simulink model "test_mdl1"  (R2023a)
settings: Solver=VariableStepAuto  StartTime=0.0  StopTime=10.0  RelTol=1e-3
(part 7 of 8)

== system test_mdl1/VehicleCAN/PCM/PowertrainData_6 ==
  BrkTot_Tq_RqFapLc : Constant  Value=0
  FapLc_B_Err : Constant  Value=0
  TrnAin_Pc_RqDrv : Constant  Value=0
  bus_creator : BusCreator  Inputs=3
  out_port : Outport
  wires:
  bus_creator/1 -> out_port/1  "test_mdl1"
  BrkTot_Tq_RqFapLc/1 -> bus_creator/1  "BrkTot_Tq_RqFapLc"
  FapLc_B_Err/1 -> bus_creator/2  "FapLc_B_Err"
  TrnAin_Pc_RqDrv/1 -> bus_creator/3  "TrnAin_Pc_RqDrv"

== system test_mdl1/VehicleCAN/PCM/PowertrainData_7 ==
  EcoCochA_Pc_Dsply : Constant  Value=0
  EcoCochCrus_Pc_Dsply : Constant  Value=0
  EcoCochDecel_Pc_Dsply : Constant  Value=0
  EcoCochIdlFuel_Pc_Dsply : Constant  Value=0
  EcoCochInstNeg_B_Dsply : Constant  Value=0
  EcoCochInst_Pc_Dsply : Constant  Value=0
  EcoCochShif_Pc_Dsply : Constant  Value=0
  bus_creator : BusCreator  Inputs=7
  out_port : Outport
  wires:
  bus_creator/1 -> out_port/1  "test_mdl1"
  EcoCochA_Pc_Dsply/1 -> bus_creator/1  "EcoCochA_Pc_Dsply"
  EcoCochCrus_Pc_Dsply/1 -> bus_creator/2  "EcoCochCrus_Pc_Dsply"
  EcoCochDecel_Pc_Dsply/1 -> bus_creator/3  "EcoCochDecel_Pc_Dsply"
  EcoCochIdlFuel_Pc_Dsply/1 -> bus_creator/4  "EcoCochIdlFuel_Pc_Dsply"
  EcoCochInstNeg_B_Dsply/1 -> bus_creator/5  "EcoCochInstNeg_B_Dsply"
  EcoCochInst_Pc_Dsply/1 -> bus_creator/6  "EcoCochInst_Pc_Dsply"
  EcoCochShif_Pc_Dsply/1 -> bus_creator/7  "EcoCochShif_Pc_Dsply"

== system test_mdl1/VehicleCAN/PCM/PowertrainData_9 ==
  AutoTowActv_B_Stat : Constant  Value=0
  AutoTowAllw_D_StatMnu : Constant  Value=0
  EngExhMdeQuiet_D2_Stat : Constant  Value=0
  GrossTrainWeight_M_Est : Constant  Value=0
  HvacCmprLim_D_Stat : Constant  Value=0
  TrailCtlPt_B_Falt : Constant  Value=0
  Veh_V_DsplyTrailCtlSet : Constant  Value=0
  WakeAlarm1_B_Typ : Constant  Value=0
  WakeAlarm1_T_Rq : Constant  Value=0
  bus_creator : BusCreator  Inputs=9
  out_port : Outport
  wires:
  bus_creator/1 -> out_port/1  "test_mdl1"
  AutoTowActv_B_Stat/1 -> bus_creator/1  "AutoTowActv_B_Stat"
  AutoTowAllw_D_StatMnu/1 -> bus_creator/2  "AutoTowAllw_D_StatMnu"
  EngExhMdeQuiet_D2_Stat/1 -> bus_creator/3  "EngExhMdeQuiet_D2_Stat"
  GrossTrainWeight_M_Est/1 -> bus_creator/4  "GrossTrainWeight_M_Est"
  HvacCmprLim_D_Stat/1 -> bus_creator/5  "HvacCmprLim_D_Stat"
  TrailCtlPt_B_Falt/1 -> bus_creator/6  "TrailCtlPt_B_Falt"
  Veh_V_DsplyTrailCtlSet/1 -> bus_creator/7  "Veh_V_DsplyTrailCtlSet"
  WakeAlarm1_B_Typ/1 -> bus_creator/8  "WakeAlarm1_B_Typ"
  WakeAlarm1_T_Rq/1 -> bus_creator/9  "WakeAlarm1_T_Rq"

== system test_mdl1/VehicleCAN/PCM/Powertrain_Data_4 ==
  BpedDrvMsgTxt_B_Dsply : Constant  Value=0
  FuelLvlWarn_D_ActlEng : Constant  Value=0
  FuelLvl_Pc_DsplyEng : Constant  Value=0
  FuelRange_L_DsplyEng : Constant  Value=0
  RearDiffOilTeWarn_B_Rq : Constant  Value=0
  RearDiffOil_Te_Actl : Constant  Value=0
  SelDrvMdePt_D_Stat : Constant  Value=0
  bus_creator : BusCreator  Inputs=7
  out_port : Outport
  wires:
  bus_creator/1 -> out_port/1  "test_mdl1"
  BpedDrvMsgTxt_B_Dsply/1 -> bus_creator/1  "BpedDrvMsgTxt_B_Dsply"
  FuelLvlWarn_D_ActlEng/1 -> bus_creator/2  "FuelLvlWarn_D_ActlEng"
  FuelLvl_Pc_DsplyEng/1 -> bus_creator/3  "FuelLvl_Pc_DsplyEng"
  FuelRange_L_DsplyEng/1 -> bus_creator/4  "FuelRange_L_DsplyEng"
  RearDiffOilTeWarn_B_Rq/1 -> bus_creator/5  "RearDiffOilTeWarn_B_Rq"
  RearDiffOil_Te_Actl/1 -> bus_creator/6  "RearDiffOil_Te_Actl"
  SelDrvMdePt_D_Stat/1 -> bus_creator/7  "SelDrvMdePt_D_Stat"

== system test_mdl1/VehicleCAN/PCM/Powertrain_Data_5 ==
  AdasLcObtclAbrt_B_Stat : Constant  Value=0
  AirDamPos_D_Stat : Constant  Value=0
  BattRgenLoChrg_D_RqEng : Constant  Value=0
  BattRgenLoDChrg_D_RqEng : Constant  Value=0
  FapLcActv_B_Stat : Constant  Value=0
  FapLcInhbt_B_Rq : Constant  Value=0
  FapLcMaxGrdAbrt_B_Stat : Constant  Value=0
  FapLcMaxGrdInhbt_B_Stat : Constant  Value=0
  FapLcObstcl_B_Stat : Constant  Value=0
  FapLcPrchgBrk_B_Rq : Constant  Value=0
  FapLcStopHold_B_Rq : Constant  Value=0
  bus_creator : BusCreator  Inputs=11
  out_port : Outport
  wires:
  bus_creator/1 -> out_port/1  "test_mdl1"
  AdasLcObtclAbrt_B_Stat/1 -> bus_creator/1  "AdasLcObtclAbrt_B_Stat"
  AirDamPos_D_Stat/1 -> bus_creator/2  "AirDamPos_D_Stat"
  BattRgenLoChrg_D_RqEng/1 -> bus_creator/3  "BattRgenLoChrg_D_RqEng"
  BattRgenLoDChrg_D_RqEng/1 -> bus_creator/4  "BattRgenLoDChrg_D_RqEng"
  FapLcActv_B_Stat/1 -> bus_creator/5  "FapLcActv_B_Stat"
  FapLcInhbt_B_Rq/1 -> bus_creator/6  "FapLcInhbt_B_Rq"
  FapLcMaxGrdAbrt_B_Stat/1 -> bus_creator/7  "FapLcMaxGrdAbrt_B_Stat"
  FapLcMaxGrdInhbt_B_Stat/1 -> bus_creator/8  "FapLcMaxGrdInhbt_B_Stat"
  FapLcObstcl_B_Stat/1 -> bus_creator/9  "FapLcObstcl_B_Stat"
  FapLcPrchgBrk_B_Rq/1 -> bus_creator/10  "FapLcPrchgBrk_B_Rq"
  FapLcStopHold_B_Rq/1 -> bus_creator/11  "FapLcStopHold_B_Rq"

== system test_mdl1/VehicleCAN/PCM/Stop_Start ==
  AutoStopPtDelta_I_Est : Constant  Value=0
  HiElPwInhbt_B_Stat : Constant  Value=0
  OdoTripVerify_L_Actl : Constant  Value=0
  StopStrtDrvMde_D_Indic : Constant  Value=0
  StopStrtIODTxt_D_Rq : Constant  Value=0
  StopStrtMsgTxt_D_Rq : Constant  Value=0
  StopStrtStdby_D_Indic : Constant  Value=0
  bus_creator : BusCreator  Inputs=7
  out_port : Outport
  wires:
  bus_creator/1 -> out_port/1  "test_mdl1"
  AutoStopPtDelta_I_Est/1 -> bus_creator/1  "AutoStopPtDelta_I_Est"
  HiElPwInhbt_B_Stat/1 -> bus_creator/2  "HiElPwInhbt_B_Stat"
  OdoTripVerify_L_Actl/1 -> bus_creator/3  "OdoTripVerify_L_Actl"
  StopStrtDrvMde_D_Indic/1 -> bus_creator/4  "StopStrtDrvMde_D_Indic"
  StopStrtIODTxt_D_Rq/1 -> bus_creator/5  "StopStrtIODTxt_D_Rq"
  StopStrtMsgTxt_D_Rq/1 -> bus_creator/6  "StopStrtMsgTxt_D_Rq"
  StopStrtStdby_D_Indic/1 -> bus_creator/7  "StopStrtStdby_D_Indic"

== system test_mdl1/VehicleCAN/PCM/TesterPhysicalResPCM ==
  TesterPhysicalResPCM : Constant  Value=0
  bus_creator : BusCreator  Inputs=1
  out_port : Outport
  wires:
  bus_creator/1 -> out_port/1  "test_mdl1"
  TesterPhysicalResPCM/1 -> bus_creator/1  "TesterPhysicalResPCM"

== system test_mdl1/VehicleCAN/PCM/TorqueDataEngFlags ==
  PrplWhlTotTqRq_No_Cnt : Constant  Value=0
  PrplWhlTotTqRq_No_Cs : Constant  Value=0
  PrplWhlTot_Tq_LimMn : Constant  Value=0
  PrplWhlTot_Tq_Rq : Constant  Value=0
  PtDrvMde_D_Stat : Constant  Value=0
  bus_creator : BusCreator  Inputs=5
  out_port : Outport
  wires:
  bus_creator/1 -> out_port/1  "test_mdl1"
  PrplWhlTotTqRq_No_Cnt/1 -> bus_creator/1  "PrplWhlTotTqRq_No_Cnt"
  PrplWhlTotTqRq_No_Cs/1 -> bus_creator/2  "PrplWhlTotTqRq_No_Cs"
  PrplWhlTot_Tq_LimMn/1 -> bus_creator/3  "PrplWhlTot_Tq_LimMn"
  PrplWhlTot_Tq_Rq/1 -> bus_creator/4  "PrplWhlTot_Tq_Rq"
  PtDrvMde_D_Stat/1 -> bus_creator/5  "PtDrvMde_D_Stat"

== system test_mdl1/VehicleCAN/PCM/TransGearData ==
  GboxOil_Te_Actl : Constant  Value=0
  GearLvrPos_D_Actl : Constant  Value=0
  SelDrvMdeSwtch_D_Stat3 : Constant  Value=0
  TrnShifActv_B_Actl : Constant  Value=0
  TrnSrvcRqd_B_Rq : Constant  Value=0
  bus_creator : BusCreator  Inputs=5
  out_port : Outport
  wires:
  bus_creator/1 -> out_port/1  "test_mdl1"
  GboxOil_Te_Actl/1 -> bus_creator/1  "GboxOil_Te_Actl"
  GearLvrPos_D_Actl/1 -> bus_creator/2  "GearLvrPos_D_Actl"
  SelDrvMdeSwtch_D_Stat3/1 -> bus_creator/3  "SelDrvMdeSwtch_D_Stat3"
  TrnShifActv_B_Actl/1 -> bus_creator/4  "TrnShifActv_B_Actl"
  TrnSrvcRqd_B_Rq/1 -> bus_creator/5  "TrnSrvcRqd_B_Rq"

== system test_mdl1/VehicleCAN/PCM/VehicleOperatingModes ==
  ElPw_D_Stat : Constant  Value=0
  ElPw_D_StatStrtStop : Constant  Value=0
  Eng_D_Stat : Constant  Value=0
  PlgActvArb_B_Actl : Constant  Value=0
  PrplWhlRgenMn_Tq_Actl : Constant  Value=0
  PrplWhlTot2_Tq_Actl : Constant  Value=0
  PwPckTq_D_Stat : Constant  Value=0
  TrnAinTq_D_Qf : Constant  Value=0
  TrnAin_Tq_Actl : Constant  Value=0
  bus_creator : BusCreator  Inputs=9
  out_port : Outport
  wires:
  bus_creator/1 -> out_port/1  "test_mdl1"
  ElPw_D_Stat/1 -> bus_creator/1  "ElPw_D_Stat"
  ElPw_D_StatStrtStop/1 -> bus_creator/2  "ElPw_D_StatStrtStop"
  Eng_D_Stat/1 -> bus_creator/3  "Eng_D_Stat"
  PlgActvArb_B_Actl/1 -> bus_creator/4  "PlgActvArb_B_Actl"
  PrplWhlRgenMn_Tq_Actl/1 -> bus_creator/5  "PrplWhlRgenMn_Tq_Actl"
  PrplWhlTot2_Tq_Actl/1 -> bus_creator/6  "PrplWhlTot2_Tq_Actl"
  PwPckTq_D_Stat/1 -> bus_creator/7  "PwPckTq_D_Stat"
  TrnAinTq_D_Qf/1 -> bus_creator/8  "TrnAinTq_D_Qf"
  TrnAin_Tq_Actl/1 -> bus_creator/9  "TrnAin_Tq_Actl"

== system test_mdl1/VehicleCAN/PCM_HEV/Cluster_HEV_Data10_FD1 ==
  Rng%ChrgAvg_L_Dsply : Constant  Value=0
  bus_creator : BusCreator  Inputs=1
  out_port : Outport
  wires:
  bus_creator/1 -> out_port/1  "test_mdl1"
  Rng%ChrgAvg_L_Dsply/1 -> bus_creator/1  "Rng%ChrgAvg_L_Dsply"

== system test_mdl1/VehicleCAN/PCM_HEV/Cluster_HEV_Data1_FD1 ==
  ChrgStat_D_Dsply : Constant  Value=0
  RgenTrip_L_Dsply : Constant  Value=0
  RgenTrip_Pc_Dsply : Constant  Value=0
  bus_creator : BusCreator  Inputs=3
  out_port : Outport
  wires:
  bus_creator/1 -> out_port/1  "test_mdl1"
  ChrgStat_D_Dsply/1 -> bus_creator/1  "ChrgStat_D_Dsply"
  RgenTrip_L_Dsply/1 -> bus_creator/2  "RgenTrip_L_Dsply"
  RgenTrip_Pc_Dsply/1 -> bus_creator/3  "RgenTrip_Pc_Dsply"

== system test_mdl1/VehicleCAN/PCM_HEV/Cluster_HEV_Data2 ==
  EffWhlLvl2_Pc_Dsply : Constant  Value=0
  EffWhlThresOn_B_Dsply : Constant  Value=0
  EffWhlThres_Pc_Dsply : Constant  Value=0
  EngActv_B_Dsply : Constant  Value=0
  EngOnMsg1_D_Dsply : Constant  Value=0
  EngOnMsg2_D_Dsply : Constant  Value=0
  EngPwLvl_Pc_Dsply : Constant  Value=0
  FuelMaintMde_D_Dsply : Constant  Value=0
  PwrFlowTxt_D_Dsply : Constant  Value=0
  bus_creator : BusCreator  Inputs=9
  out_port : Outport
  wires:
  bus_creator/1 -> out_port/1  "test_mdl1"
  EffWhlLvl2_Pc_Dsply/1 -> bus_creator/1  "EffWhlLvl2_Pc_Dsply"
  EffWhlThresOn_B_Dsply/1 -> bus_creator/2  "EffWhlThresOn_B_Dsply"
  EffWhlThres_Pc_Dsply/1 -> bus_creator/3  "EffWhlThres_Pc_Dsply"
  EngActv_B_Dsply/1 -> bus_creator/4  "EngActv_B_Dsply"
  EngOnMsg1_D_Dsply/1 -> bus_creator/5  "EngOnMsg1_D_Dsply"
  EngOnMsg2_D_Dsply/1 -> bus_creator/6  "EngOnMsg2_D_Dsply"
  EngPwLvl_Pc_Dsply/1 -> bus_creator/7  "EngPwLvl_Pc_Dsply"
  FuelMaintMde_D_Dsply/1 -> bus_creator/8  "FuelMaintMde_D_Dsply"
  PwrFlowTxt_D_Dsply/1 -> bus_creator/9  "PwrFlowTxt_D_Dsply"

== system test_mdl1/VehicleCAN/PCM_HEV/Cluster_HEV_Data3_FD1 ==
  EffRgenThres_Pc_Dsply : Constant  Value=0
  EngMdeMsgTxt_D_Rq : Constant  Value=0
  Rng%ChrgInst_L_Dsply : Constant  Value=0
  bus_creator : BusCreator  Inputs=3
  out_port : Outport
  wires:
  bus_creator/1 -> out_port/1  "test_mdl1"
  EffRgenThres_Pc_Dsply/1 -> bus_creator/1  "EffRgenThres_Pc_Dsply"
  EngMdeMsgTxt_D_Rq/1 -> bus_creator/2  "EngMdeMsgTxt_D_Rq"
  Rng%ChrgInst_L_Dsply/1 -> bus_creator/3  "Rng%ChrgInst_L_Dsply"

== system test_mdl1/VehicleCAN/PCM_HEV/Cluster_HEV_Data5 ==
  HybMdeStat_D_Dsply : Constant  Value=0
  PlgActvArb_B_Dsply : Constant  Value=0
  bus_creator : BusCreator  Inputs=2
  out_port : Outport
  wires:
  bus_creator/1 -> out_port/1  "test_mdl1"
  HybMdeStat_D_Dsply/1 -> bus_creator/1  "HybMdeStat_D_Dsply"
  PlgActvArb_B_Dsply/1 -> bus_creator/2  "PlgActvArb_B_Dsply"

== system test_mdl1/VehicleCAN/PCM_HEV/DCACA_Data4 ==
  DcacElPw_D_Stat : Constant  Value=0
  DcacEngOnMsgTxt_D_Rq : Constant  Value=0
  DcacFaltMsgTxt_D_Rq : Constant  Value=0
  DcacGfciTest_B_Rq : Constant  Value=0
  DcacHw_D_Confg : Constant  Value=0
  DcacLedCtl_D_Rq : Constant  Value=0
  DcacLoFuelMsgTxt_D_Rq : Constant  Value=0
  DcacOn_B_Rq : Constant  Value=0
  DcacOut1_Pw_Dsply : Constant  Value=0
  DcacOut2_Pw_Dsply : Constant  Value=0
  DcacOut_Pw_DsplyMx : Constant  Value=0
  DcacSys_B_Falt : Constant  Value=0
  PwBedPnlEnbl_B_Rq : Constant  Value=0
  bus_creator : BusCreator  Inputs=13
  out_port : Outport
  wires:
  bus_creator/1 -> out_port/1  "test_mdl1"
  DcacElPw_D_Stat/1 -> bus_creator/1  "DcacElPw_D_Stat"
  DcacEngOnMsgTxt_D_Rq/1 -> bus_creator/2  "DcacEngOnMsgTxt_D_Rq"
  DcacFaltMsgTxt_D_Rq/1 -> bus_creator/3  "DcacFaltMsgTxt_D_Rq"
  DcacGfciTest_B_Rq/1 -> bus_creator/4  "DcacGfciTest_B_Rq"
  DcacHw_D_Confg/1 -> bus_creator/5  "DcacHw_D_Confg"
  DcacLedCtl_D_Rq/1 -> bus_creator/6  "DcacLedCtl_D_Rq"
  DcacLoFuelMsgTxt_D_Rq/1 -> bus_creator/7  "DcacLoFuelMsgTxt_D_Rq"
  DcacOn_B_Rq/1 -> bus_creator/8  "DcacOn_B_Rq"
  DcacOut1_Pw_Dsply/1 -> bus_creator/9  "DcacOut1_Pw_Dsply"
  DcacOut2_Pw_Dsply/1 -> bus_creator/10  "DcacOut2_Pw_Dsply"
  DcacOut_Pw_DsplyMx/1 -> bus_creator/11  "DcacOut_Pw_DsplyMx"
  DcacSys_B_Falt/1 -> bus_creator/12  "DcacSys_B_Falt"
  PwBedPnlEnbl_B_Rq/1 -> bus_creator/13  "PwBedPnlEnbl_B_Rq"

== system test_mdl1/VehicleCAN/PCM_HEV/EngBrakeData ==
  AccEngStat_D_Actl : Constant  Value=0
  AccStopMde_D_Rq : Constant  Value=0
  BPedDrvAppl_D_QF : Constant  Value=0
  BpedDrvAppl_D_Actl : Constant  Value=0
  CcMde_D_Actl : Constant  Value=0
  CcOvrrdActv_B_Actl : Constant  Value=0
  CcStat_D_Actl : Constant  Value=0
  CmbbDeny_B_ActlPrpl : Constant  Value=0
  CmbbEngTqMn_B_Actl : Constant  Value=0
  EngAout_N_MnAllw : Constant  Value=0
  PrplTqMnSat_B_Actl : Constant  Value=0
  Veh_V_DsplyCcSet : Constant  Value=0
  bus_creator : BusCreator  Inputs=12
  out_port : Outport
  wires:
  bus_creator/1 -> out_port/1  "test_mdl1"
  AccEngStat_D_Actl/1 -> bus_creator/1  "AccEngStat_D_Actl"
  AccStopMde_D_Rq/1 -> bus_creator/2  "AccStopMde_D_Rq"
  BPedDrvAppl_D_QF/1 -> bus_creator/3  "BPedDrvAppl_D_QF"
  BpedDrvAppl_D_Actl/1 -> bus_creator/4  "BpedDrvAppl_D_Actl"
  CcMde_D_Actl/1 -> bus_creator/5  "CcMde_D_Actl"
  CcOvrrdActv_B_Actl/1 -> bus_creator/6  "CcOvrrdActv_B_Actl"
  CcStat_D_Actl/1 -> bus_creator/7  "CcStat_D_Actl"
  CmbbDeny_B_ActlPrpl/1 -> bus_creator/8  "CmbbDeny_B_ActlPrpl"
  CmbbEngTqMn_B_Actl/1 -> bus_creator/9  "CmbbEngTqMn_B_Actl"
  EngAout_N_MnAllw/1 -> bus_creator/10  "EngAout_N_MnAllw"
  PrplTqMnSat_B_Actl/1 -> bus_creator/11  "PrplTqMnSat_B_Actl"
  Veh_V_DsplyCcSet/1 -> bus_creator/12  "Veh_V_DsplyCcSet"

== system test_mdl1/VehicleCAN/PCM_HEV/EngVehicleSpThrottle ==
  ApedPosPcActl_D_Qf : Constant  Value=0
  ApedPosPcActl_No_Cnt : Constant  Value=0
  ApedPosPcActl_No_Cs : Constant  Value=0
  ApedPos_PcRate_ActlArb : Constant  Value=0
  ApedPos_Pc_ActlArb : Constant  Value=0
  EngAout3_N_Actl : Constant  Value=0
  EngAoutNActl_D_QF : Constant  Value=0
  EngAout_N_Actl : Constant  Value=0
  bus_creator : BusCreator  Inputs=8
  out_port : Outport
  wires:
  bus_creator/1 -> out_port/1  "test_mdl1"
  ApedPosPcActl_D_Qf/1 -> bus_creator/1  "ApedPosPcActl_D_Qf"
  ApedPosPcActl_No_Cnt/1 -> bus_creator/2  "ApedPosPcActl_No_Cnt"
  ApedPosPcActl_No_Cs/1 -> bus_creator/3  "ApedPosPcActl_No_Cs"
  ApedPos_PcRate_ActlArb/1 -> bus_creator/4  "ApedPos_PcRate_ActlArb"
  ApedPos_Pc_ActlArb/1 -> bus_creator/5  "ApedPos_Pc_ActlArb"
  EngAout3_N_Actl/1 -> bus_creator/6  "EngAout3_N_Actl"
  EngAoutNActl_D_QF/1 -> bus_creator/7  "EngAoutNActl_D_QF"
  EngAout_N_Actl/1 -> bus_creator/8  "EngAout_N_Actl"

== system test_mdl1/VehicleCAN/PCM_HEV/EngVehicleSpThrottle2 ==
  GearRvrse_D_Actl : Constant  Value=0
  StrtrMtrCtlMsgTxt_D2_Rq : Constant  Value=0
  StrtrMtrCtlMsgTxt_D_Rq : Constant  Value=0
  StrtrMtrDlyStrt_B_Stat : Constant  Value=0
  VehVActlEng_D_Qf : Constant  Value=0
  VehVActlEng_No_Cnt : Constant  Value=0
  VehVActlEng_No_Cs : Constant  Value=0
  VehVTrlrAid_B_Avail : Constant  Value=0
  Veh_V_ActlEng : Constant  Value=0
  Veh_V_RqCcSet : Constant  Value=0
  bus_creator : BusCreator  Inputs=10
  out_port : Outport
  wires:
  bus_creator/1 -> out_port/1  "test_mdl1"
  GearRvrse_D_Actl/1 -> bus_creator/1  "GearRvrse_D_Actl"
  StrtrMtrCtlMsgTxt_D2_Rq/1 -> bus_creator/2  "StrtrMtrCtlMsgTxt_D2_Rq"
  StrtrMtrCtlMsgTxt_D_Rq/1 -> bus_creator/3  "StrtrMtrCtlMsgTxt_D_Rq"
  StrtrMtrDlyStrt_B_Stat/1 -> bus_creator/4  "StrtrMtrDlyStrt_B_Stat"
  VehVActlEng_D_Qf/1 -> bus_creator/5  "VehVActlEng_D_Qf"
  VehVActlEng_No_Cnt/1 -> bus_creator/6  "VehVActlEng_No_Cnt"
  VehVActlEng_No_Cs/1 -> bus_creator/7  "VehVActlEng_No_Cs"
  VehVTrlrAid_B_Avail/1 -> bus_creator/8  "VehVTrlrAid_B_Avail"
  Veh_V_ActlEng/1 -> bus_creator/9  "Veh_V_ActlEng"
  Veh_V_RqCcSet/1 -> bus_creator/10  "Veh_V_RqCcSet"

== system test_mdl1/VehicleCAN/PCM_HEV/EngineClimateData ==
  AirAmbTe_D_Qf : Constant  Value=0
  AirAmb_P_Actl : Constant  Value=0
  AirAmb_Te_Actl : Constant  Value=0
  AirAmb_Te_ActlFilt : Constant  Value=0
  AslChime_B_Rq : Constant  Value=0
  AslIconDsply_D_Rq : Constant  Value=0
  DynoMde_B_Cmd : Constant  Value=0
  EcssLamp_D_RqDsply : Constant  Value=0
  EngAout_Aa_Actl : Constant  Value=0
  GasPrtc_D_RqDsply : Constant  Value=0
  HvacHtrCore2_Te_Actl : Constant  Value=0
  bus_creator : BusCreator  Inputs=11
  out_port : Outport
  wires:
  bus_creator/1 -> out_port/1  "test_mdl1"
  AirAmbTe_D_Qf/1 -> bus_creator/1  "AirAmbTe_D_Qf"
  AirAmb_P_Actl/1 -> bus_creator/2  "AirAmb_P_Actl"
  AirAmb_Te_Actl/1 -> bus_creator/3  "AirAmb_Te_Actl"
  AirAmb_Te_ActlFilt/1 -> bus_creator/4  "AirAmb_Te_ActlFilt"
  AslChime_B_Rq/1 -> bus_creator/5  "AslChime_B_Rq"
  AslIconDsply_D_Rq/1 -> bus_creator/6  "AslIconDsply_D_Rq"
  DynoMde_B_Cmd/1 -> bus_creator/7  "DynoMde_B_Cmd"
  EcssLamp_D_RqDsply/1 -> bus_creator/8  "EcssLamp_D_RqDsply"
  EngAout_Aa_Actl/1 -> bus_creator/9  "EngAout_Aa_Actl"
  GasPrtc_D_RqDsply/1 -> bus_creator/10  "GasPrtc_D_RqDsply"
  HvacHtrCore2_Te_Actl/1 -> bus_creator/11  "HvacHtrCore2_Te_Actl"

== system test_mdl1/VehicleCAN/PCM_HEV/EngineData_1 ==
  SeatWorkSrfc_B_Falt : Constant  Value=0
  TrnIpcDsplyGear_D_Actl : Constant  Value=0
  TrnIpcDsplyGear_D_Stat : Constant  Value=0
  TrnIpcDsplyMde_D_Actl : Constant  Value=0
  TrnIpcDsplyMde_D_Stat : Constant  Value=0
  TrnIpcDsplyRng2_D_Actl : Constant  Value=0
  TrnIpcDsplyRng_D_Stat : Constant  Value=0
  bus_creator : BusCreator  Inputs=7
  out_port : Outport
  wires:
  bus_creator/1 -> out_port/1  "test_mdl1"
  SeatWorkSrfc_B_Falt/1 -> bus_creator/1  "SeatWorkSrfc_B_Falt"
  TrnIpcDsplyGear_D_Actl/1 -> bus_creator/2  "TrnIpcDsplyGear_D_Actl"
  TrnIpcDsplyGear_D_Stat/1 -> bus_creator/3  "TrnIpcDsplyGear_D_Stat"
  TrnIpcDsplyMde_D_Actl/1 -> bus_creator/4  "TrnIpcDsplyMde_D_Actl"
  TrnIpcDsplyMde_D_Stat/1 -> bus_creator/5  "TrnIpcDsplyMde_D_Stat"
  TrnIpcDsplyRng2_D_Actl/1 -> bus_creator/6  "TrnIpcDsplyRng2_D_Actl"
  TrnIpcDsplyRng_D_Stat/1 -> bus_creator/7  "TrnIpcDsplyRng_D_Stat"

== system test_mdl1/VehicleCAN/PCM_HEV/EngineData_6 ==
  EngClntTe_D_Qf : Constant  Value=0
  EngClnt_Te_Actl : Constant  Value=0
  EngGoutLss_Tq_Est : Constant  Value=0
  EngOil_Te_Actl : Constant  Value=0
  EngOvrhtMitgActv_D_Ind : Constant  Value=0
  bus_creator : BusCreator  Inputs=5
  out_port : Outport
  wires:
  bus_creator/1 -> out_port/1  "test_mdl1"
  EngClntTe_D_Qf/1 -> bus_creator/1  "EngClntTe_D_Qf"
  EngClnt_Te_Actl/1 -> bus_creator/2  "EngClnt_Te_Actl"
  EngGoutLss_Tq_Est/1 -> bus_creator/3  "EngGoutLss_Tq_Est"
  EngOil_Te_Actl/1 -> bus_creator/4  "EngOil_Te_Actl"
  EngOvrhtMitgActv_D_Ind/1 -> bus_creator/5  "EngOvrhtMitgActv_D_Ind"

== system test_mdl1/VehicleCAN/PCM_HEV/EngineData_7 ==
  AirCondClutch_B_Stats : Constant  Value=0
  AirCondRec_B_Rq : Constant  Value=0
  EngOilLife_Pc_Actl : Constant  Value=0
  EngSrvcRqd_B_Rq : Constant  Value=0
  FuelFillInlet_B_Dsply : Constant  Value=0
  FuelFilterLamp_B_Dsply : Constant  Value=0
  FuelFlw_Vl_Dsply : Constant  Value=0
  HvacAirFullOut_B_Rq : Constant  Value=0
  OdoCount : Constant  Value=0
  bus_creator : BusCreator  Inputs=9
  out_port : Outport
  wires:
  bus_creator/1 -> out_port/1  "test_mdl1"
  AirCondClutch_B_Stats/1 -> bus_creator/1  "AirCondClutch_B_Stats"
  AirCondRec_B_Rq/1 -> bus_creator/2  "AirCondRec_B_Rq"
  EngOilLife_Pc_Actl/1 -> bus_creator/3  "EngOilLife_Pc_Actl"
  EngSrvcRqd_B_Rq/1 -> bus_creator/4  "EngSrvcRqd_B_Rq"
  FuelFillInlet_B_Dsply/1 -> bus_creator/5  "FuelFillInlet_B_Dsply"
  FuelFilterLamp_B_Dsply/1 -> bus_creator/6  "FuelFilterLamp_B_Dsply"
  FuelFlw_Vl_Dsply/1 -> bus_creator/7  "FuelFlw_Vl_Dsply"
  HvacAirFullOut_B_Rq/1 -> bus_creator/8  "HvacAirFullOut_B_Rq"
  OdoCount/1 -> bus_creator/9  "OdoCount"

== system test_mdl1/VehicleCAN/PCM_HEV/Engine_Clutch_Data ==
  CluPdlPosPcMeas_D_Qf : Constant  Value=0
  CluPdlPos_Pc_Meas : Constant  Value=0
  CluPdl_PcRate_Actl : Constant  Value=0
  EngAoutIdl_N_Ntrl : Constant  Value=0
  EngAout_N_Dsply : Constant  Value=0
  bus_creator : BusCreator  Inputs=5
  out_port : Outport
  wires:
  bus_creator/1 -> out_port/1  "test_mdl1"
  CluPdlPosPcMeas_D_Qf/1 -> bus_creator/1  "CluPdlPosPcMeas_D_Qf"
  CluPdlPos_Pc_Meas/1 -> bus_creator/2  "CluPdlPos_Pc_Meas"
  CluPdl_PcRate_Actl/1 -> bus_creator/3  "CluPdl_PcRate_Actl"
  EngAoutIdl_N_Ntrl/1 -> bus_creator/4  "EngAoutIdl_N_Ntrl"
  EngAout_N_Dsply/1 -> bus_creator/5  "EngAout_N_Dsply"

== system test_mdl1/VehicleCAN/PCM_HEV/Gear_Shift_by_Wire_3 ==
  GearSelLck_D_Rq : Constant  Value=0
  PrkBrkActv_D_RqTrnGear : Constant  Value=0
  TrnCmdCnt_B_Actl : Constant  Value=0
  TrnCmdState_B_Actl : Constant  Value=0
  TrnDtpCmd_D_Actl : Constant  Value=0
  TrnGearCmd_No_Cnt : Constant  Value=0
  TrnGearCmd_No_Cs : Constant  Value=0
  TrnGearCmd_Pc_ActlPt : Constant  Value=0
  TrnGearMsgTxt_D_Rq : Constant  Value=0
  TrnGearNtmAllow_B_Stat : Constant  Value=0
  TrnGear_D_RqPt : Constant  Value=0
  TrnLvrV_D_Rq : Constant  Value=0
  TrnNtrlTowCmd_D_Actl : Constant  Value=0
  TrnSbwSysHlth_D_Actl : Constant  Value=0
  TrnValidGear_D_Cnfm : Constant  Value=0
  bus_creator : BusCreator  Inputs=15
  out_port : Outport
  wires:
  bus_creator/1 -> out_port/1  "test_mdl1"
  GearSelLck_D_Rq/1 -> bus_creator/1  "GearSelLck_D_Rq"
  PrkBrkActv_D_RqTrnGear/1 -> bus_creator/2  "PrkBrkActv_D_RqTrnGear"
  TrnCmdCnt_B_Actl/1 -> bus_creator/3  "TrnCmdCnt_B_Actl"
  TrnCmdState_B_Actl/1 -> bus_creator/4  "TrnCmdState_B_Actl"
  TrnDtpCmd_D_Actl/1 -> bus_creator/5  "TrnDtpCmd_D_Actl"
  TrnGearCmd_No_Cnt/1 -> bus_creator/6  "TrnGearCmd_No_Cnt"
  TrnGearCmd_No_Cs/1 -> bus_creator/7  "TrnGearCmd_No_Cs"
  TrnGearCmd_Pc_ActlPt/1 -> bus_creator/8  "TrnGearCmd_Pc_ActlPt"
  TrnGearMsgTxt_D_Rq/1 -> bus_creator/9  "TrnGearMsgTxt_D_Rq"
  TrnGearNtmAllow_B_Stat/1 -> bus_creator/10  "TrnGearNtmAllow_B_Stat"
  TrnGear_D_RqPt/1 -> bus_creator/11  "TrnGear_D_RqPt"
  TrnLvrV_D_Rq/1 -> bus_creator/12  "TrnLvrV_D_Rq"
  TrnNtrlTowCmd_D_Actl/1 -> bus_creator/13  "TrnNtrlTowCmd_D_Actl"
  TrnSbwSysHlth_D_Actl/1 -> bus_creator/14  "TrnSbwSysHlth_D_Actl"
  TrnValidGear_D_Cnfm/1 -> bus_creator/15  "TrnValidGear_D_Cnfm"

== system test_mdl1/VehicleCAN/PCM_HEV/Global_PATS_TargetInfo ==
  bus_creator : BusCreator  Inputs=3
  immoTarget1Cmd : Constant  Value=0
  immoTarget1Data : Constant  Value=0
  immoTarget1Status : Constant  Value=0
  out_port : Outport
  wires:
  bus_creator/1 -> out_port/1  "test_mdl1"
  immoTarget1Cmd/1 -> bus_creator/1  "immoTarget1Cmd"
  immoTarget1Data/1 -> bus_creator/2  "immoTarget1Data"
  immoTarget1Status/1 -> bus_creator/3  "immoTarget1Status"

== system test_mdl1/VehicleCAN/PCM_HEV/HEV_Powertrain_Data ==
  HtrnWarnLamp_B_Dsply : Constant  Value=0
  HybPwLimOn_B_Stat : Constant  Value=0
  PwPckTqRdy_B_Dsply : Constant  Value=0
  bus_creator : BusCreator  Inputs=3
  out_port : Outport
  wires:
  bus_creator/1 -> out_port/1  "test_mdl1"
  HtrnWarnLamp_B_Dsply/1 -> bus_creator/1  "HtrnWarnLamp_B_Dsply"
  HybPwLimOn_B_Stat/1 -> bus_creator/2  "HybPwLimOn_B_Stat"
  PwPckTqRdy_B_Dsply/1 -> bus_creator/3  "PwPckTqRdy_B_Dsply"

== system test_mdl1/VehicleCAN/PCM_HEV/HEV_Powertrain_Data2 ==
  BattTracCnnct_D_Rq : Constant  Value=0
  PrplTqMnRgen_B_Actl : Constant  Value=0
  WhlDirAvgDrv_D_Actl : Constant  Value=0
  bus_creator : BusCreator  Inputs=3
  out_port : Outport
  wires:
  bus_creator/1 -> out_port/1  "test_mdl1"
  BattTracCnnct_D_Rq/1 -> bus_creator/1  "BattTracCnnct_D_Rq"
  PrplTqMnRgen_B_Actl/1 -> bus_creator/2  "PrplTqMnRgen_B_Actl"
  WhlDirAvgDrv_D_Actl/1 -> bus_creator/3  "WhlDirAvgDrv_D_Actl"

== system test_mdl1/VehicleCAN/PCM_HEV/HEV_Powertrain_Data6 ==
  BattTracDiagClr_B_Stat : Constant  Value=0
  DcdcOn_B_Rq : Constant  Value=0
  EngTeHi_B_Actl : Constant  Value=0
  ULoBattSpprtSustn_B_Rq : Constant  Value=0
  VehElEff_No_Avg : Constant  Value=0
  bus_creator : BusCreator  Inputs=5
  out_port : Outport
  wires:
  bus_creator/1 -> out_port/1  "test_mdl1"
  BattTracDiagClr_B_Stat/1 -> bus_creator/1  "BattTracDiagClr_B_Stat"
  DcdcOn_B_Rq/1 -> bus_creator/2  "DcdcOn_B_Rq"
  EngTeHi_B_Actl/1 -> bus_creator/3  "EngTeHi_B_Actl"
  ULoBattSpprtSustn_B_Rq/1 -> bus_creator/4  "ULoBattSpprtSustn_B_Rq"
  VehElEff_No_Avg/1 -> bus_creator/5  "VehElEff_No_Avg"

== system test_mdl1/VehicleCAN/PCM_HEV/HEV_Powertrain_Data7_FD1 ==
  PwFlwBattClimt_B_Dsply : Constant  Value=0
  PwFlwBatt_D_Dsply : Constant  Value=0
  PwFlwFuelBatt_B_Dsply : Constant  Value=0
  PwFlwFuelClimt_B_Dsply : Constant  Value=0
  PwFlwFuelDrv_D_Dsply : Constant  Value=0
  RngImpctClim_L_Dsply : Constant  Value=0
  RngImpctDrv_L_Dsply : Constant  Value=0
  VehElEffAvg_No_Dsply : Constant  Value=0
  bus_creator : BusCreator  Inputs=8
  out_port : Outport
  wires:
  bus_creator/1 -> out_port/1  "test_mdl1"
  PwFlwBattClimt_B_Dsply/1 -> bus_creator/1  "PwFlwBattClimt_B_Dsply"
  PwFlwBatt_D_Dsply/1 -> bus_creator/2  "PwFlwBatt_D_Dsply"
  PwFlwFuelBatt_B_Dsply/1 -> bus_creator/3  "PwFlwFuelBatt_B_Dsply"
  PwFlwFuelClimt_B_Dsply/1 -> bus_creator/4  "PwFlwFuelClimt_B_Dsply"
  PwFlwFuelDrv_D_Dsply/1 -> bus_creator/5  "PwFlwFuelDrv_D_Dsply"
  RngImpctClim_L_Dsply/1 -> bus_creator/6  "RngImpctClim_L_Dsply"
  RngImpctDrv_L_Dsply/1 -> bus_creator/7  "RngImpctDrv_L_Dsply"
  VehElEffAvg_No_Dsply/1 -> bus_creator/8  "VehElEffAvg_No_Dsply"

== system test_mdl1/VehicleCAN/PCM_HEV/HEV_Powertrain_Data8_FD1 ==
  ElVehLaterMde_D_Stat : Constant  Value=0
  ElVehNowMde_D_Stat : Constant  Value=0
  bus_creator : BusCreator  Inputs=2
  out_port : Outport
  wires:
  bus_creator/1 -> out_port/1  "test_mdl1"
  ElVehLaterMde_D_Stat/1 -> bus_creator/1  "ElVehLaterMde_D_Stat"
  ElVehNowMde_D_Stat/1 -> bus_creator/2  "ElVehNowMde_D_Stat"

== system test_mdl1/VehicleCAN/PCM_HEV/MtrTrac_Data2_FD1 ==
  ChrgStat_D_ActlMntr : Constant  Value=0
  HybVehMde_D_ActlMntr : Constant  Value=0
  Inv1Ain_I_ActlMntr : Constant  Value=0
  Mtr2State_D_ActlMntr : Constant  Value=0
  VehElRnge_L_Dsply : Constant  Value=0
  bus_creator : BusCreator  Inputs=5
  out_port : Outport
  wires:
  bus_creator/1 -> out_port/1  "test_mdl1"
  ChrgStat_D_ActlMntr/1 -> bus_creator/1  "ChrgStat_D_ActlMntr"
  HybVehMde_D_ActlMntr/1 -> bus_creator/2  "HybVehMde_D_ActlMntr"
  Inv1Ain_I_ActlMntr/1 -> bus_creator/3  "Inv1Ain_I_ActlMntr"
  Mtr2State_D_ActlMntr/1 -> bus_creator/4  "Mtr2State_D_ActlMntr"
  VehElRnge_L_Dsply/1 -> bus_creator/5  "VehElRnge_L_Dsply"

== system test_mdl1/VehicleCAN/PCM_HEV/OTAPhysPCMtoGWM_ECG ==
  OTAPhysPCMtoGWM_ECG : Constant  Value=0
  bus_creator : BusCreator  Inputs=1
  out_port : Outport
  wires:
  bus_creator/1 -> out_port/1  "test_mdl1"
  OTAPhysPCMtoGWM_ECG/1 -> bus_creator/1  "OTAPhysPCMtoGWM_ECG"

== system test_mdl1/VehicleCAN/PCM_HEV/PARSEDPhysPCMtoGWM_ECG ==
  PARSEDPhysPCMtoGWM_ECG : Constant  Value=0
  bus_creator : BusCreator  Inputs=1
  out_port : Outport
  wires:
  bus_creator/1 -> out_port/1  "test_mdl1"
  PARSEDPhysPCMtoGWM_ECG/1 -> bus_creator/1  "PARSEDPhysPCMtoGWM_ECG"

== system test_mdl1/VehicleCAN/PCM_HEV/PARSEDPushPCMtoGWM_ECG ==
  PARSEDPushPCMtoGWM_ECG : Constant  Value=0
  bus_creator : BusCreator  Inputs=1
  out_port : Outport
  wires:
  bus_creator/1 -> out_port/1  "test_mdl1"
  PARSEDPushPCMtoGWM_ECG/1 -> bus_creator/1  "PARSEDPushPCMtoGWM_ECG"

== system test_mdl1/VehicleCAN/PCM_HEV/PCM_AutoSar_NetworkMgmt ==
  PCM_AutoSarNMControl : Constant  Value=0
  PCM_AutoSarNMNodeId : Constant  Value=0
  PCM_AutoSarNMReserved{1..4} (4 alike) : Constant  Value=0
  PCM_GWNMProxy : Constant  Value=0
  PCM_GWOnBoardTester : Constant  Value=0
  bus_creator : BusCreator  Inputs=8
  out_port : Outport
  wires:
  bus_creator/1 -> out_port/1  "test_mdl1"
  PCM_AutoSarNMControl/1 -> bus_creator/1  "PCM_AutoSarNMControl"
  PCM_AutoSarNMNodeId/1 -> bus_creator/2  "PCM_AutoSarNMNodeId"
  PCM_AutoSarNMReserved1/1 -> bus_creator/3  "PCM_AutoSarNMReserved1"
  PCM_AutoSarNMReserved2/1 -> bus_creator/4  "PCM_AutoSarNMReserved2"
  PCM_AutoSarNMReserved3/1 -> bus_creator/5  "PCM_AutoSarNMReserved3"
  PCM_AutoSarNMReserved4/1 -> bus_creator/6  "PCM_AutoSarNMReserved4"
  PCM_GWNMProxy/1 -> bus_creator/7  "PCM_GWNMProxy"
  PCM_GWOnBoardTester/1 -> bus_creator/8  "PCM_GWOnBoardTester"

== system test_mdl1/VehicleCAN/PCM_HEV/PCM_Rapid_Data_Response_1 ==
  UUDTPCMResponse1 : Constant  Value=0
  bus_creator : BusCreator  Inputs=1
  out_port : Outport
  wires:
  bus_creator/1 -> out_port/1  "test_mdl1"
  UUDTPCMResponse1/1 -> bus_creator/1  "UUDTPCMResponse1"

== system test_mdl1/VehicleCAN/PCM_HEV/PCM_Rapid_Data_Response_2 ==
  UUDTPCMResponse2 : Constant  Value=0
  bus_creator : BusCreator  Inputs=1
  out_port : Outport
  wires:
  bus_creator/1 -> out_port/1  "test_mdl1"
  UUDTPCMResponse2/1 -> bus_creator/1  "UUDTPCMResponse2"

== system test_mdl1/VehicleCAN/PCM_HEV/PowertrainData_1 ==
  AirCondFluidHi_P_Actl : Constant  Value=0
  CoolantFanStepAct : Constant  Value=0
  ECMMILRequest : Constant  Value=0
  EngIdlShutDown_D_Stat : Constant  Value=0
  EngIdlShutDwnTxt_D_Rq : Constant  Value=0
  FUEL_ALCOHOL_PERCNT : Constant  Value=0
  FohEng_D_Rq : Constant  Value=0
  OilPressureWarning : Constant  Value=0
  TrnTotLss_Tq_Est : Constant  Value=0
  TrnTotTq_Rt_Est : Constant  Value=0
  VehVLimActv_B_Actl : Constant  Value=0
  VehVLimStat_D_Actl : Constant  Value=0
  bus_creator : BusCreator  Inputs=12
  out_port : Outport
  wires:
  bus_creator/1 -> out_port/1  "test_mdl1"
  AirCondFluidHi_P_Actl/1 -> bus_creator/1  "AirCondFluidHi_P_Actl"
  CoolantFanStepAct/1 -> bus_creator/2  "CoolantFanStepAct"
  ECMMILRequest/1 -> bus_creator/3  "ECMMILRequest"
  EngIdlShutDown_D_Stat/1 -> bus_creator/4  "EngIdlShutDown_D_Stat"
  EngIdlShutDwnTxt_D_Rq/1 -> bus_creator/5  "EngIdlShutDwnTxt_D_Rq"
  FUEL_ALCOHOL_PERCNT/1 -> bus_creator/6  "FUEL_ALCOHOL_PERCNT"
  FohEng_D_Rq/1 -> bus_creator/7  "FohEng_D_Rq"
  OilPressureWarning/1 -> bus_creator/8  "OilPressureWarning"
  TrnTotLss_Tq_Est/1 -> bus_creator/9  "TrnTotLss_Tq_Est"
  TrnTotTq_Rt_Est/1 -> bus_creator/10  "TrnTotTq_Rt_Est"
  VehVLimActv_B_Actl/1 -> bus_creator/11  "VehVLimActv_B_Actl"
  VehVLimStat_D_Actl/1 -> bus_creator/12  "VehVLimStat_D_Actl"

== system test_mdl1/VehicleCAN/PCM_HEV/PowertrainData_10 ==
  GearEngag_D_Actl : Constant  Value=0
  GearLvr_D_ActlDrv : Constant  Value=0
  GearPos_D_Actl : Constant  Value=0
  GearPos_D_Trg : Constant  Value=0
  GearPos_No_Cnt : Constant  Value=0
  GearPos_No_Cs : Constant  Value=0
  TrnIgnOffDly_T_Rq : Constant  Value=0
  TrnPrkSys_D_Actl : Constant  Value=0
  TrnRng_D_Rq : Constant  Value=0
  bus_creator : BusCreator  Inputs=9
  out_port : Outport
  wires:
  bus_creator/1 -> out_port/1  "test_mdl1"
  GearEngag_D_Actl/1 -> bus_creator/1  "GearEngag_D_Actl"
  GearLvr_D_ActlDrv/1 -> bus_creator/2  "GearLvr_D_ActlDrv"
  GearPos_D_Actl/1 -> bus_creator/3  "GearPos_D_Actl"
  GearPos_D_Trg/1 -> bus_creator/4  "GearPos_D_Trg"
  GearPos_No_Cnt/1 -> bus_creator/5  "GearPos_No_Cnt"
  GearPos_No_Cs/1 -> bus_creator/6  "GearPos_No_Cs"
  TrnIgnOffDly_T_Rq/1 -> bus_creator/7  "TrnIgnOffDly_T_Rq"
  TrnPrkSys_D_Actl/1 -> bus_creator/8  "TrnPrkSys_D_Actl"
  TrnRng_D_Rq/1 -> bus_creator/9  "TrnRng_D_Rq"

== system test_mdl1/VehicleCAN/PCM_HEV/PowertrainData_2 ==
  ApedPos_Pc_ActlDiag : Constant  Value=0
  EngAirIn_Te_Actl : Constant  Value=0
  EngClnt_Te_ActlDiag : Constant  Value=0
  EngLoad_Pc_CalcDiag : Constant  Value=0
  EngMsgTxt_D_Rq : Constant  Value=0
  GrllShtrPos_B_Falt : Constant  Value=0
  GrllShtrPos_D_Cmd : Constant  Value=0
  IsaOffst_D_Stat : Constant  Value=0
  ObdWarmUp_B_Complt : Constant  Value=0
  SlMde_D_RqDsply : Constant  Value=0
  SlMde_D_Stat : Constant  Value=0
  bus_creator : BusCreator  Inputs=11
  out_port : Outport
  wires:
  bus_creator/1 -> out_port/1  "test_mdl1"
  ApedPos_Pc_ActlDiag/1 -> bus_creator/1  "ApedPos_Pc_ActlDiag"
  EngAirIn_Te_Actl/1 -> bus_creator/2  "EngAirIn_Te_Actl"
  EngClnt_Te_ActlDiag/1 -> bus_creator/3  "EngClnt_Te_ActlDiag"
  EngLoad_Pc_CalcDiag/1 -> bus_creator/4  "EngLoad_Pc_CalcDiag"
  EngMsgTxt_D_Rq/1 -> bus_creator/5  "EngMsgTxt_D_Rq"
  GrllShtrPos_B_Falt/1 -> bus_creator/6  "GrllShtrPos_B_Falt"
  GrllShtrPos_D_Cmd/1 -> bus_creator/7  "GrllShtrPos_D_Cmd"
  IsaOffst_D_Stat/1 -> bus_creator/8  "IsaOffst_D_Stat"
  ObdWarmUp_B_Complt/1 -> bus_creator/9  "ObdWarmUp_B_Complt"
  SlMde_D_RqDsply/1 -> bus_creator/10  "SlMde_D_RqDsply"
  SlMde_D_Stat/1 -> bus_creator/11  "SlMde_D_Stat"

== system test_mdl1/VehicleCAN/PCM_HEV/PowertrainData_3 ==
  BattULoChrg_U_Cmd : Constant  Value=0
  ElLoadCtl_D_Rq : Constant  Value=0
  EngMnfld_P_Actl : Constant  Value=0
  FuelPumpPwr_B_Rq : Constant  Value=0
  bus_creator : BusCreator  Inputs=4
  out_port : Outport
  wires:
  bus_creator/1 -> out_port/1  "test_mdl1"
  BattULoChrg_U_Cmd/1 -> bus_creator/1  "BattULoChrg_U_Cmd"
  ElLoadCtl_D_Rq/1 -> bus_creator/2  "ElLoadCtl_D_Rq"
  EngMnfld_P_Actl/1 -> bus_creator/3  "EngMnfld_P_Actl"
  FuelPumpPwr_B_Rq/1 -> bus_creator/4  "FuelPumpPwr_B_Rq"

== system test_mdl1/VehicleCAN/PCM_HEV/PowertrainData_6 ==
  BrkTot_Tq_RqFapLc : Constant  Value=0
  FapLc_B_Err : Constant  Value=0
  TrnAin_Pc_RqDrv : Constant  Value=0
  bus_creator : BusCreator  Inputs=3
  out_port : Outport
  wires:
  bus_creator/1 -> out_port/1  "test_mdl1"
  BrkTot_Tq_RqFapLc/1 -> bus_creator/1  "BrkTot_Tq_RqFapLc"
  FapLc_B_Err/1 -> bus_creator/2  "FapLc_B_Err"
  TrnAin_Pc_RqDrv/1 -> bus_creator/3  "TrnAin_Pc_RqDrv"

== system test_mdl1/VehicleCAN/PCM_HEV/PowertrainData_7 ==
  EcoCochA_Pc_Dsply : Constant  Value=0
  EcoCochCrus_Pc_Dsply : Constant  Value=0
  EcoCochDecel_Pc_Dsply : Constant  Value=0
  EcoCochIdlFuel_Pc_Dsply : Constant  Value=0
  EcoCochInstNeg_B_Dsply : Constant  Value=0
  EcoCochInst_Pc_Dsply : Constant  Value=0
  EcoCochShif_Pc_Dsply : Constant  Value=0
  bus_creator : BusCreator  Inputs=7
  out_port : Outport
  wires:
  bus_creator/1 -> out_port/1  "test_mdl1"
  EcoCochA_Pc_Dsply/1 -> bus_creator/1  "EcoCochA_Pc_Dsply"
  EcoCochCrus_Pc_Dsply/1 -> bus_creator/2  "EcoCochCrus_Pc_Dsply"
  EcoCochDecel_Pc_Dsply/1 -> bus_creator/3  "EcoCochDecel_Pc_Dsply"
  EcoCochIdlFuel_Pc_Dsply/1 -> bus_creator/4  "EcoCochIdlFuel_Pc_Dsply"
  EcoCochInstNeg_B_Dsply/1 -> bus_creator/5  "EcoCochInstNeg_B_Dsply"
  EcoCochInst_Pc_Dsply/1 -> bus_creator/6  "EcoCochInst_Pc_Dsply"
  EcoCochShif_Pc_Dsply/1 -> bus_creator/7  "EcoCochShif_Pc_Dsply"

== system test_mdl1/VehicleCAN/PCM_HEV/PowertrainData_9 ==
  AutoTowActv_B_Stat : Constant  Value=0
  AutoTowAllw_D_StatMnu : Constant  Value=0
  EngExhMdeQuiet_D2_Stat : Constant  Value=0
  GrossTrainWeight_M_Est : Constant  Value=0
  HvacCmprLim_D_Stat : Constant  Value=0
  TrailCtlPt_B_Falt : Constant  Value=0
  Veh_V_DsplyTrailCtlSet : Constant  Value=0
  WakeAlarm1_B_Typ : Constant  Value=0
  WakeAlarm1_T_Rq : Constant  Value=0
  bus_creator : BusCreator  Inputs=9
  out_port : Outport
  wires:
  bus_creator/1 -> out_port/1  "test_mdl1"
  AutoTowActv_B_Stat/1 -> bus_creator/1  "AutoTowActv_B_Stat"
  AutoTowAllw_D_StatMnu/1 -> bus_creator/2  "AutoTowAllw_D_StatMnu"
  EngExhMdeQuiet_D2_Stat/1 -> bus_creator/3  "EngExhMdeQuiet_D2_Stat"
  GrossTrainWeight_M_Est/1 -> bus_creator/4  "GrossTrainWeight_M_Est"
  HvacCmprLim_D_Stat/1 -> bus_creator/5  "HvacCmprLim_D_Stat"
  TrailCtlPt_B_Falt/1 -> bus_creator/6  "TrailCtlPt_B_Falt"
  Veh_V_DsplyTrailCtlSet/1 -> bus_creator/7  "Veh_V_DsplyTrailCtlSet"
  WakeAlarm1_B_Typ/1 -> bus_creator/8  "WakeAlarm1_B_Typ"
  WakeAlarm1_T_Rq/1 -> bus_creator/9  "WakeAlarm1_T_Rq"

== system test_mdl1/VehicleCAN/PCM_HEV/Powertrain_Data_4 ==
  BpedDrvMsgTxt_B_Dsply : Constant  Value=0
  FuelLvlWarn_D_ActlEng : Constant  Value=0
  FuelLvl_Pc_DsplyEng : Constant  Value=0
  FuelRange_L_DsplyEng : Constant  Value=0
  RearDiffOilTeWarn_B_Rq : Constant  Value=0
  RearDiffOil_Te_Actl : Constant  Value=0
  SelDrvMdePt_D_Stat : Constant  Value=0
  bus_creator : BusCreator  Inputs=7
  out_port : Outport
  wires:
  bus_creator/1 -> out_port/1  "test_mdl1"
  BpedDrvMsgTxt_B_Dsply/1 -> bus_creator/1  "BpedDrvMsgTxt_B_Dsply"
  FuelLvlWarn_D_ActlEng/1 -> bus_creator/2  "FuelLvlWarn_D_ActlEng"
  FuelLvl_Pc_DsplyEng/1 -> bus_creator/3  "FuelLvl_Pc_DsplyEng"
  FuelRange_L_DsplyEng/1 -> bus_creator/4  "FuelRange_L_DsplyEng"
  RearDiffOilTeWarn_B_Rq/1 -> bus_creator/5  "RearDiffOilTeWarn_B_Rq"
  RearDiffOil_Te_Actl/1 -> bus_creator/6  "RearDiffOil_Te_Actl"
  SelDrvMdePt_D_Stat/1 -> bus_creator/7  "SelDrvMdePt_D_Stat"

== system test_mdl1/VehicleCAN/PCM_HEV/Powertrain_Data_5 ==
  AdasLcObtclAbrt_B_Stat : Constant  Value=0
  AirDamPos_D_Stat : Constant  Value=0
  BattRgenLoChrg_D_RqEng : Constant  Value=0
  BattRgenLoDChrg_D_RqEng : Constant  Value=0
  FapLcActv_B_Stat : Constant  Value=0
  FapLcInhbt_B_Rq : Constant  Value=0
  FapLcMaxGrdAbrt_B_Stat : Constant  Value=0
  FapLcMaxGrdInhbt_B_Stat : Constant  Value=0
  FapLcObstcl_B_Stat : Constant  Value=0
  FapLcPrchgBrk_B_Rq : Constant  Value=0
  FapLcStopHold_B_Rq : Constant  Value=0
  bus_creator : BusCreator  Inputs=11
  out_port : Outport
  wires:
  bus_creator/1 -> out_port/1  "test_mdl1"
  AdasLcObtclAbrt_B_Stat/1 -> bus_creator/1  "AdasLcObtclAbrt_B_Stat"
  AirDamPos_D_Stat/1 -> bus_creator/2  "AirDamPos_D_Stat"
  BattRgenLoChrg_D_RqEng/1 -> bus_creator/3  "BattRgenLoChrg_D_RqEng"
  BattRgenLoDChrg_D_RqEng/1 -> bus_creator/4  "BattRgenLoDChrg_D_RqEng"
  FapLcActv_B_Stat/1 -> bus_creator/5  "FapLcActv_B_Stat"
  FapLcInhbt_B_Rq/1 -> bus_creator/6  "FapLcInhbt_B_Rq"
  FapLcMaxGrdAbrt_B_Stat/1 -> bus_creator/7  "FapLcMaxGrdAbrt_B_Stat"
  FapLcMaxGrdInhbt_B_Stat/1 -> bus_creator/8  "FapLcMaxGrdInhbt_B_Stat"
  FapLcObstcl_B_Stat/1 -> bus_creator/9  "FapLcObstcl_B_Stat"
  FapLcPrchgBrk_B_Rq/1 -> bus_creator/10  "FapLcPrchgBrk_B_Rq"
  FapLcStopHold_B_Rq/1 -> bus_creator/11  "FapLcStopHold_B_Rq"

== system test_mdl1/VehicleCAN/PCM_HEV/Stop_Start ==
  AutoStopPtDelta_I_Est : Constant  Value=0
  HiElPwInhbt_B_Stat : Constant  Value=0
  OdoTripVerify_L_Actl : Constant  Value=0
  StopStrtDrvMde_D_Indic : Constant  Value=0
  StopStrtIODTxt_D_Rq : Constant  Value=0
  StopStrtMsgTxt_D_Rq : Constant  Value=0
  StopStrtStdby_D_Indic : Constant  Value=0
  bus_creator : BusCreator  Inputs=7
  out_port : Outport
  wires:
  bus_creator/1 -> out_port/1  "test_mdl1"
  AutoStopPtDelta_I_Est/1 -> bus_creator/1  "AutoStopPtDelta_I_Est"
  HiElPwInhbt_B_Stat/1 -> bus_creator/2  "HiElPwInhbt_B_Stat"
  OdoTripVerify_L_Actl/1 -> bus_creator/3  "OdoTripVerify_L_Actl"
  StopStrtDrvMde_D_Indic/1 -> bus_creator/4  "StopStrtDrvMde_D_Indic"
  StopStrtIODTxt_D_Rq/1 -> bus_creator/5  "StopStrtIODTxt_D_Rq"
  StopStrtMsgTxt_D_Rq/1 -> bus_creator/6  "StopStrtMsgTxt_D_Rq"
  StopStrtStdby_D_Indic/1 -> bus_creator/7  "StopStrtStdby_D_Indic"

== system test_mdl1/VehicleCAN/PCM_HEV/TesterPhysicalResPCM ==
  TesterPhysicalResPCM : Constant  Value=0
  bus_creator : BusCreator  Inputs=1
  out_port : Outport
  wires:
  bus_creator/1 -> out_port/1  "test_mdl1"
  TesterPhysicalResPCM/1 -> bus_creator/1  "TesterPhysicalResPCM"

== system test_mdl1/VehicleCAN/PCM_HEV/TorqueDataEngFlags ==
  PrplWhlTotTqRq_No_Cnt : Constant  Value=0
  PrplWhlTotTqRq_No_Cs : Constant  Value=0
  PrplWhlTot_Tq_LimMn : Constant  Value=0
  PrplWhlTot_Tq_Rq : Constant  Value=0
  PtDrvMde_D_Stat : Constant  Value=0
  bus_creator : BusCreator  Inputs=5
  out_port : Outport
  wires:
  bus_creator/1 -> out_port/1  "test_mdl1"
  PrplWhlTotTqRq_No_Cnt/1 -> bus_creator/1  "PrplWhlTotTqRq_No_Cnt"
  PrplWhlTotTqRq_No_Cs/1 -> bus_creator/2  "PrplWhlTotTqRq_No_Cs"
  PrplWhlTot_Tq_LimMn/1 -> bus_creator/3  "PrplWhlTot_Tq_LimMn"
  PrplWhlTot_Tq_Rq/1 -> bus_creator/4  "PrplWhlTot_Tq_Rq"
  PtDrvMde_D_Stat/1 -> bus_creator/5  "PtDrvMde_D_Stat"

== system test_mdl1/VehicleCAN/PCM_HEV/TransGearData ==
  GboxOil_Te_Actl : Constant  Value=0
  GearLvrPos_D_Actl : Constant  Value=0
  SelDrvMdeSwtch_D_Stat3 : Constant  Value=0
  TrnShifActv_B_Actl : Constant  Value=0
  TrnSrvcRqd_B_Rq : Constant  Value=0
  bus_creator : BusCreator  Inputs=5
  out_port : Outport
  wires:
  bus_creator/1 -> out_port/1  "test_mdl1"
  GboxOil_Te_Actl/1 -> bus_creator/1  "GboxOil_Te_Actl"
  GearLvrPos_D_Actl/1 -> bus_creator/2  "GearLvrPos_D_Actl"
  SelDrvMdeSwtch_D_Stat3/1 -> bus_creator/3  "SelDrvMdeSwtch_D_Stat3"
  TrnShifActv_B_Actl/1 -> bus_creator/4  "TrnShifActv_B_Actl"
  TrnSrvcRqd_B_Rq/1 -> bus_creator/5  "TrnSrvcRqd_B_Rq"

== system test_mdl1/VehicleCAN/PCM_HEV/VehicleOperatingModes ==
  ElPw_D_Stat : Constant  Value=0
  ElPw_D_StatStrtStop : Constant  Value=0
  Eng_D_Stat : Constant  Value=0
  PlgActvArb_B_Actl : Constant  Value=0
  PrplWhlRgenMn_Tq_Actl : Constant  Value=0
  PrplWhlTot2_Tq_Actl : Constant  Value=0
  PwPckTq_D_Stat : Constant  Value=0
  TrnAinTq_D_Qf : Constant  Value=0
  TrnAin_Tq_Actl : Constant  Value=0
  bus_creator : BusCreator  Inputs=9
  out_port : Outport
  wires:
  bus_creator/1 -> out_port/1  "test_mdl1"
  ElPw_D_Stat/1 -> bus_creator/1  "ElPw_D_Stat"
  ElPw_D_StatStrtStop/1 -> bus_creator/2  "ElPw_D_StatStrtStop"
  Eng_D_Stat/1 -> bus_creator/3  "Eng_D_Stat"
  PlgActvArb_B_Actl/1 -> bus_creator/4  "PlgActvArb_B_Actl"
  PrplWhlRgenMn_Tq_Actl/1 -> bus_creator/5  "PrplWhlRgenMn_Tq_Actl"
  PrplWhlTot2_Tq_Actl/1 -> bus_creator/6  "PrplWhlTot2_Tq_Actl"
  PwPckTq_D_Stat/1 -> bus_creator/7  "PwPckTq_D_Stat"
  TrnAinTq_D_Qf/1 -> bus_creator/8  "TrnAinTq_D_Qf"
  TrnAin_Tq_Actl/1 -> bus_creator/9  "TrnAin_Tq_Actl"

== system test_mdl1/VehicleCAN/PSCM/EPAS_INFO ==
  DrvSteActv_B_Stat : Constant  Value=0
  DrvSte_Tq_Actl : Constant  Value=0
  EPAS_Failure : Constant  Value=0
  SAPPAngleControlStat{1..6} (6 alike) : Constant  Value=0
  SteMdule_D_Stat : Constant  Value=0
  SteMdule_I_Est : Constant  Value=0
  SteMdule_U_Meas : Constant  Value=0
  SteeringColumnTorque : Constant  Value=0
  TrlrHitchLamp_D_Rqst : Constant  Value=0
  VehVTrlrAid_B_Rq : Constant  Value=0
  Veh_V_RqMxTrlrAid : Constant  Value=0
  bus_creator : BusCreator  Inputs=16
  out_port : Outport
  wires:
  bus_creator/1 -> out_port/1  "test_mdl1"
  DrvSteActv_B_Stat/1 -> bus_creator/1  "DrvSteActv_B_Stat"
  DrvSte_Tq_Actl/1 -> bus_creator/2  "DrvSte_Tq_Actl"
  EPAS_Failure/1 -> bus_creator/3  "EPAS_Failure"
  SAPPAngleControlStat1/1 -> bus_creator/4  "SAPPAngleControlStat1"
  SAPPAngleControlStat2/1 -> bus_creator/5  "SAPPAngleControlStat2"
  SAPPAngleControlStat3/1 -> bus_creator/6  "SAPPAngleControlStat3"
  SAPPAngleControlStat4/1 -> bus_creator/7  "SAPPAngleControlStat4"
  SAPPAngleControlStat5/1 -> bus_creator/8  "SAPPAngleControlStat5"
  SAPPAngleControlStat6/1 -> bus_creator/9  "SAPPAngleControlStat6"
  SteMdule_D_Stat/1 -> bus_creator/10  "SteMdule_D_Stat"
  SteMdule_I_Est/1 -> bus_creator/11  "SteMdule_I_Est"
  SteMdule_U_Meas/1 -> bus_creator/12  "SteMdule_U_Meas"
  SteeringColumnTorque/1 -> bus_creator/13  "SteeringColumnTorque"
  TrlrHitchLamp_D_Rqst/1 -> bus_creator/14  "TrlrHitchLamp_D_Rqst"
  VehVTrlrAid_B_Rq/1 -> bus_creator/15  "VehVTrlrAid_B_Rq"
  Veh_V_RqMxTrlrAid/1 -> bus_creator/16  "Veh_V_RqMxTrlrAid"

== system test_mdl1/VehicleCAN/PSCM/Lane_Assist_Data3_FD1 ==
  LaActAvail_D_Actl : Constant  Value=0
  LaActDeny_B_Actl : Constant  Value=0
  LaHandsOff_B_Actl : Constant  Value=0
  LatCtlCpbltyDStat_No_Cnt : Constant  Value=0
  LatCtlCpbltyDStat_No_Cs : Constant  Value=0
  LatCtlCpblty_D_Stat : Constant  Value=0
  LatCtlLim_D_Stat : Constant  Value=0
  LatCtlSte_D_Stat : Constant  Value=0
  LsmcBrkDecelEnbl_D_Rq : Constant  Value=0
  LsmcBrk_Tq_Rq : Constant  Value=0
  TjaHandsOnCnfdnc_B_Est : Constant  Value=0
  TrlrAn_An_TrgtCalc : Constant  Value=0
  bus_creator : BusCreator  Inputs=12
  out_port : Outport
  wires:
  bus_creator/1 -> out_port/1  "test_mdl1"
  LaActAvail_D_Actl/1 -> bus_creator/1  "LaActAvail_D_Actl"
  LaActDeny_B_Actl/1 -> bus_creator/2  "LaActDeny_B_Actl"
  LaHandsOff_B_Actl/1 -> bus_creator/3  "LaHandsOff_B_Actl"
  LatCtlCpbltyDStat_No_Cnt/1 -> bus_creator/4  "LatCtlCpbltyDStat_No_Cnt"
  LatCtlCpbltyDStat_No_Cs/1 -> bus_creator/5  "LatCtlCpbltyDStat_No_Cs"
  LatCtlCpblty_D_Stat/1 -> bus_creator/6  "LatCtlCpblty_D_Stat"
  LatCtlLim_D_Stat/1 -> bus_creator/7  "LatCtlLim_D_Stat"
  LatCtlSte_D_Stat/1 -> bus_creator/8  "LatCtlSte_D_Stat"
  LsmcBrkDecelEnbl_D_Rq/1 -> bus_creator/9  "LsmcBrkDecelEnbl_D_Rq"
  LsmcBrk_Tq_Rq/1 -> bus_creator/10  "LsmcBrk_Tq_Rq"
  TjaHandsOnCnfdnc_B_Est/1 -> bus_creator/11  "TjaHandsOnCnfdnc_B_Est"
  TrlrAn_An_TrgtCalc/1 -> bus_creator/12  "TrlrAn_An_TrgtCalc"

== system test_mdl1/VehicleCAN/PSCM/PSCM_AutoSar_NetwrkMgmt ==
  PSCM_AutoSarNMControl : Constant  Value=0
  PSCM_AutoSarNMNodeId : Constant  Value=0
  PSCM_AutoSarNMReserved{1..4} (4 alike) : Constant  Value=0
  PSCM_GWNMProxy : Constant  Value=0
  PSCM_GWOnBoardTester : Constant  Value=0
  bus_creator : BusCreator  Inputs=8
  out_port : Outport
  wires:
  bus_creator/1 -> out_port/1  "test_mdl1"
  PSCM_AutoSarNMControl/1 -> bus_creator/1  "PSCM_AutoSarNMControl"
  PSCM_AutoSarNMNodeId/1 -> bus_creator/2  "PSCM_AutoSarNMNodeId"
  PSCM_AutoSarNMReserved1/1 -> bus_creator/3  "PSCM_AutoSarNMReserved1"
  PSCM_AutoSarNMReserved2/1 -> bus_creator/4  "PSCM_AutoSarNMReserved2"
  PSCM_AutoSarNMReserved3/1 -> bus_creator/5  "PSCM_AutoSarNMReserved3"
  PSCM_AutoSarNMReserved4/1 -> bus_creator/6  "PSCM_AutoSarNMReserved4"
  PSCM_GWNMProxy/1 -> bus_creator/7  "PSCM_GWNMProxy"
  PSCM_GWOnBoardTester/1 -> bus_creator/8  "PSCM_GWOnBoardTester"

== system test_mdl1/VehicleCAN/PSCM/SteeringPinion_Data ==
  StePinAn_No_Cnt : Constant  Value=0
  StePinAn_No_Cs : Constant  Value=0
  StePinCompAnEst_D_Qf : Constant  Value=0
  StePinComp_An_Est : Constant  Value=0
  StePinRelInit_An_Sns : Constant  Value=0
  StePw_B_Rq : Constant  Value=0
  bus_creator : BusCreator  Inputs=6
  out_port : Outport
  wires:
  bus_creator/1 -> out_port/1  "test_mdl1"
  StePinAn_No_Cnt/1 -> bus_creator/1  "StePinAn_No_Cnt"
  StePinAn_No_Cs/1 -> bus_creator/2  "StePinAn_No_Cs"
  StePinCompAnEst_D_Qf/1 -> bus_creator/3  "StePinCompAnEst_D_Qf"
  StePinComp_An_Est/1 -> bus_creator/4  "StePinComp_An_Est"
  StePinRelInit_An_Sns/1 -> bus_creator/5  "StePinRelInit_An_Sns"
  StePw_B_Rq/1 -> bus_creator/6  "StePw_B_Rq"

== system test_mdl1/VehicleCAN/PSCM/TesterPhysicalResPSCM ==
  TesterPhysicalResPSCM : Constant  Value=0
  bus_creator : BusCreator  Inputs=1
  out_port : Outport
  wires:
  bus_creator/1 -> out_port/1  "test_mdl1"
  TesterPhysicalResPSCM/1 -> bus_creator/1  "TesterPhysicalResPSCM"

== system test_mdl1/VehicleCAN/PSCM/TrailerAid_Data2 ==
  EsaOn_B_Stat : Constant  Value=0
  HitchToTrlrAxle_L_Calc : Constant  Value=0
  SelDrvMdeSte_D_Stat : Constant  Value=0
  TrlrAidEnbl_D2_Stat : Constant  Value=0
  TrlrAidMsgTxt_D2_Rq : Constant  Value=0
  TrlrAidSetup_D2_Stat : Constant  Value=0
  TrlrAidTrgtId_No_Rq : Constant  Value=0
  TrlrAidTrlrId_No_Rq : Constant  Value=0
  TrlrAnOffst_An2_Calc : Constant  Value=0
  TrlrAn_An_MxCalc : Constant  Value=0
  TrlrAn_An_WarnCalc : Constant  Value=0
  bus_creator : BusCreator  Inputs=11
  out_port : Outport
  wires:
  bus_creator/1 -> out_port/1  "test_mdl1"
  EsaOn_B_Stat/1 -> bus_creator/1  "EsaOn_B_Stat"
  HitchToTrlrAxle_L_Calc/1 -> bus_creator/2  "HitchToTrlrAxle_L_Calc"
  SelDrvMdeSte_D_Stat/1 -> bus_creator/3  "SelDrvMdeSte_D_Stat"
  TrlrAidEnbl_D2_Stat/1 -> bus_creator/4  "TrlrAidEnbl_D2_Stat"
  TrlrAidMsgTxt_D2_Rq/1 -> bus_creator/5  "TrlrAidMsgTxt_D2_Rq"
  TrlrAidSetup_D2_Stat/1 -> bus_creator/6  "TrlrAidSetup_D2_Stat"
  TrlrAidTrgtId_No_Rq/1 -> bus_creator/7  "TrlrAidTrgtId_No_Rq"
  TrlrAidTrlrId_No_Rq/1 -> bus_creator/8  "TrlrAidTrlrId_No_Rq"
  TrlrAnOffst_An2_Calc/1 -> bus_creator/9  "TrlrAnOffst_An2_Calc"
  TrlrAn_An_MxCalc/1 -> bus_creator/10  "TrlrAn_An_MxCalc"
  TrlrAn_An_WarnCalc/1 -> bus_creator/11  "TrlrAn_An_WarnCalc"

== system test_mdl1/VehicleCAN/SOBDMC_HPCM_FD1/AC_Compressor_Req_FD1 ==
  ElCmprEnbl_B_Rq : Constant  Value=0
  ElCmpr_N_Rq : Constant  Value=0
  bus_creator : BusCreator  Inputs=2
  out_port : Outport
  wires:
  bus_creator/1 -> out_port/1  "test_mdl1"
  ElCmprEnbl_B_Rq/1 -> bus_creator/1  "ElCmprEnbl_B_Rq"
  ElCmpr_N_Rq/1 -> bus_creator/2  "ElCmpr_N_Rq"

== system test_mdl1/VehicleCAN/SOBDMC_HPCM_FD1/ChargeSettings_FD1 ==
  ChrgLocIdCurnt_D_Sav : Constant  Value=0
  ChrgLocIdUnsAck_B_Stat : Constant  Value=0
  ChrgNowEnbl_B_Saved : Constant  Value=0
  ChrgPrflWkdy_No_Actl : Constant  Value=0
  ChrgPrflWknd_No_Actl : Constant  Value=0
  ChrgProgIdSaved_D_Stat : Constant  Value=0
  ChrgToPcWkdySav_D_Stat : Constant  Value=0
  ChrgToPcWkndSav_D_Stat : Constant  Value=0
  bus_creator : BusCreator  Inputs=8
  out_port : Outport
  wires:
  bus_creator/1 -> out_port/1  "test_mdl1"
  ChrgLocIdCurnt_D_Sav/1 -> bus_creator/1  "ChrgLocIdCurnt_D_Sav"
  ChrgLocIdUnsAck_B_Stat/1 -> bus_creator/2  "ChrgLocIdUnsAck_B_Stat"
  ChrgNowEnbl_B_Saved/1 -> bus_creator/3  "ChrgNowEnbl_B_Saved"
  ChrgPrflWkdy_No_Actl/1 -> bus_creator/4  "ChrgPrflWkdy_No_Actl"
  ChrgPrflWknd_No_Actl/1 -> bus_creator/5  "ChrgPrflWknd_No_Actl"
  ChrgProgIdSaved_D_Stat/1 -> bus_creator/6  "ChrgProgIdSaved_D_Stat"
  ChrgToPcWkdySav_D_Stat/1 -> bus_creator/7  "ChrgToPcWkdySav_D_Stat"
  ChrgToPcWkndSav_D_Stat/1 -> bus_creator/8  "ChrgToPcWkndSav_D_Stat"

== system test_mdl1/VehicleCAN/SOBDMC_HPCM_FD1/Cluster_HEV_Data1_FD1 ==
  ChrgStat_D_Dsply : Constant  Value=0
  RgenTrip_L_Dsply : Constant  Value=0
  RgenTrip_Pc_Dsply : Constant  Value=0
  bus_creator : BusCreator  Inputs=3
  out_port : Outport
  wires:
  bus_creator/1 -> out_port/1  "test_mdl1"
  ChrgStat_D_Dsply/1 -> bus_creator/1  "ChrgStat_D_Dsply"
  RgenTrip_L_Dsply/1 -> bus_creator/2  "RgenTrip_L_Dsply"
  RgenTrip_Pc_Dsply/1 -> bus_creator/3  "RgenTrip_Pc_Dsply"
